simulink model "power_3pfault_generate_testdata"  (R2017b)
settings: Solver=FixedStepDiscrete  StartTime=0.0  StopTime=0.2  FixedStep=Ts  RelTol=1e-4  EnableMultiTasking=on
PreLoadFcn:
  | Ts=50e-6;
InitFcn:
  | Ts=50e-6;
undefined symbols (not defined in the file or in its folder): D1, Delta
libraries: powerlib x23
Description:
  | Copyright 2008-2017 The MathWorks, Inc.
settings Model: ExtModeTrigMode=oneshot  ExtModeArmWhenConnect=off  ExtModeAutoUpdateStatusClock=off  Creator=MathWorks  LastModifiedBy=estheim
settings DataIOCC: SaveFormat=Array  SignalLoggingSaveFormat=ModelDataLogs  SignalLoggingName=sigsOut
settings OptimizationCC: BlockReduction=off  BooleanDataType=off  ExpressionDepthLimit=2147483647  InitFltsAndDblsToZero=on  EfficientMapNaN2IntZero=off  LifeSpan=inf
settings DebuggingCC: UnderspecifiedInitializationDetection=Classic  MergeDetectMultiDrivingBlocksExec=none  CheckExecutionContextPreStartOutputMsg=on  CheckExecutionContextRuntimeOutputMsg=on  SignalResolutionControl=TryResolveAllWithWarning  MultiTaskDSMMsg=warning  MultiTaskCondExecSysMsg=none  FcnCallInpInsideContextMsg=warning  UnconnectedInputMsg=none  UnconnectedOutputMsg=none  StateNameClashWarn=warning  SFUnexpectedBacktrackingDiag=warning  SFNoUnconditionalDefaultTransitionDiag=warning  SFExecutionAtInitializationDiag=none
settings HardwareCC: ProdBitPerPointer=32  ProdBitPerSizeT=32  ProdBitPerPtrDiffT=32  ProdLargestAtomicFloat=None  ProdIntDivRoundTo=Undefined  ProdEndianess=Unspecified  ProdWordSize=32  ProdHWDeviceType=Specified  TargetUnknown=on
settings ModelReferenceCC: PropagateSignalLabelsOutOfModel=off
settings CodeAppCC: StateflowObjectComments=on
settings GRTTargetCC: TargetLangStandard=C89/C90 (ANSI)  GeneratePreprocessorConditionals=Disable all  CombineOutputUpdateFcns=off  GRTInterface=on
settings ConfigComp: CovMetricSettings=dw  CovHtmlReporting=on  CovSaveCumulativeToWorkspaceVar=on  CovSaveSingleToWorkspaceVar=on  CovExternalEMLEnable=off  CovSFcnEnable=off
settings SimscapeCC: SimscapeNormalizeSystem=off

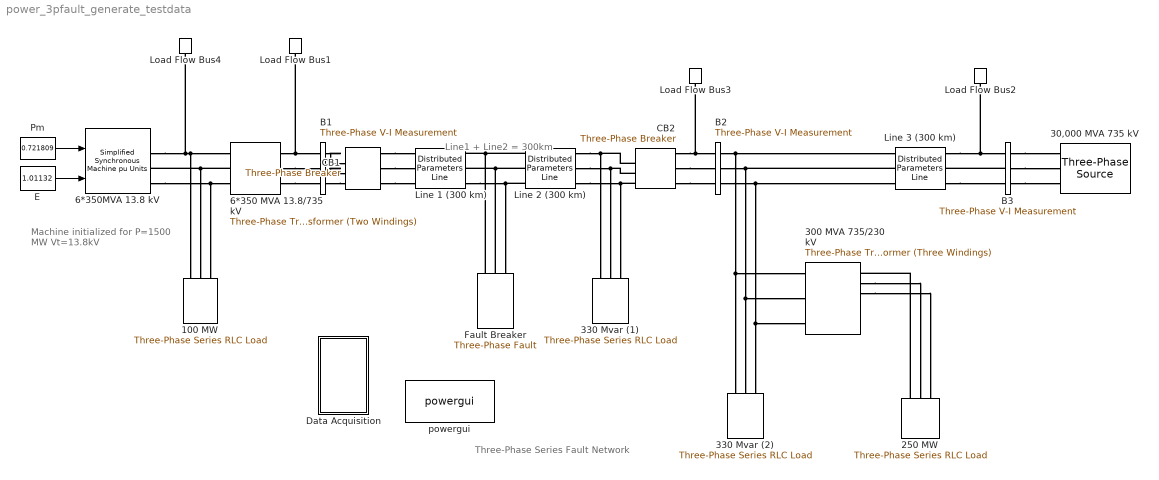
== system power_3pfault_generate_testdata ==
  note: Line1 + Line2 = 300km
  note: Machine initialized for
      |  P=1500 MW
      |  Vt=13.8kV
  note: Three-Phase Series Fault Network
  100 MW : powerlib/Elements/Three-Phase Series RLC Load  LConnTagsString=A|B|C  Configuration=Y (grounded)  NominalVoltage=13.8e3  Vabc=[1e3 1e3 1e3]  Vabcp=[1e3 1e3 1e3]  NominalFrequency=60  UnbalancedPower=off  ActivePower=100000000  InductivePower=0  CapacitivePower=0  Pabc=[10e3 9e3 11e3]  QLabc=[100 90 110]  QCabc=[100 90 110]  Pabcp=[10e3 9e3 11e3]  QLabcp=[100 90 110]  QCabcp=[100 90 110]  Measurements=None  LoadType=constant Z
  250 MW : powerlib/Elements/Three-Phase Series RLC Load  LConnTagsString=A|B|C  Configuration=Y (grounded)  NominalVoltage=230e3  Vabc=[1e3 1e3 1e3]  Vabcp=[1e3 1e3 1e3]  NominalFrequency=60  UnbalancedPower=off  ActivePower=250000000  InductivePower=0  CapacitivePower=0  Pabc=[10e3 9e3 11e3]  QLabc=[100 90 110]  QCabc=[100 90 110]  Pabcp=[10e3 9e3 11e3]  QLabcp=[100 90 110]  QCabcp=[100 90 110]  Measurements=None  LoadType=constant Z
  30,000 MVA 735 kV : powerlib/Electrical Sources/Three-Phase Source  InternalConnection=Yg  VoltagePhases=off  Voltage=(735000)*0.98865  PhaseAngle=-2.0892  Voltage_phases=[25e3 25e3 25e3]/sqrt(3)  PhaseAngles_phases=[0 -120 +120]  Frequency=60  NonIdealSource=on  SpecifyImpedance=on  Resistance=735^2/30000/10  Inductance=735^2/30000/377  ShortCircuitLevel=30000e6  BaseVoltage=735e3  XRratio=10  BusType=swing  Pref=0  Qref=0  Prefabc=[10e3, 10e3, 10e3]  Qrefabc=[0, 0, 0]  Qmin=-Inf  Qmax=Inf
  300 MVA 735/230 kV : powerlib/Elements/Three-Phase Transformer (Three Windings)  Winding1Connection=Yg  Winding2Connection=Yg  Winding3Connection=Delta (D1)  CoreType=Three single-phase transformers  SetSaturation=on  Hysteresis=off  DataFile='hysteresis'  SetInitialFlux=off  Measurements=None  UNITS=pu  NominalPower=[ 300e6 , 60 ]  Winding1=[ 735e3 , 0.002 , 0.15 ]  Winding2=[ 230e3 , 0.002 , 0 ]  Winding3=[ 25e3 , 0.05 , 0.20 ]  Rm=500  Lm=1000  L0=0.5  Saturation="[  0,0  ;  0.0012,1.2  ;  1.0,1.45 ]"  InitialFluxes=[-1.00775342585712 0.407388050044642 0.600365375812479]  MoreParameters=on  BreakLoop=on  DataType=off  TransfoNumber=0
      settings: AttributesFormatString=\n  SourceProductName=Simscape Power Systems  SourceProductBaseCode=PS
  330 Mvar (1) : powerlib/Elements/Three-Phase Series RLC Load  LConnTagsString=A|B|C  Configuration=Y (grounded)  NominalVoltage=735e3  Vabc=[1e3 1e3 1e3]  Vabcp=[1e3 1e3 1e3]  NominalFrequency=60  UnbalancedPower=off  ActivePower=1320000  InductivePower=330e6  CapacitivePower=0  Pabc=[10e3 9e3 11e3]  QLabc=[100 90 110]  QCabc=[100 90 110]  Pabcp=[10e3 9e3 11e3]  QLabcp=[100 90 110]  QCabcp=[100 90 110]  Measurements=None  LoadType=constant Z
  "330 Mvar (2) " : powerlib/Elements/Three-Phase Series RLC Load  LConnTagsString=A|B|C  Configuration=Y (grounded)  NominalVoltage=735e3  Vabc=[1e3 1e3 1e3]  Vabcp=[1e3 1e3 1e3]  NominalFrequency=60  UnbalancedPower=off  ActivePower=1320000  InductivePower=330e6  CapacitivePower=0  Pabc=[10e3 9e3 11e3]  QLabc=[100 90 110]  QCabc=[100 90 110]  Pabcp=[10e3 9e3 11e3]  QLabcp=[100 90 110]  QCabcp=[100 90 110]  Measurements=None  LoadType=constant Z
  6*350 MVA 13.8/735 kV : powerlib/Elements/Three-Phase Transformer (Two Windings)  Winding1Connection=Delta (D1)  Winding2Connection=Yg  CoreType=Three single-phase transformers  SetSaturation=off  Hysteresis=off  DataFile='hysteresis'  SetInitialFlux=off  Measurements=None  UNITS=pu  NominalPower=[ 6*350e6 , 60 ]  Winding1=[ 13.8e3 , 0.002 , 0.08 ]  Winding2=[ 735e3 , 0.002 , 0.08 ]  Rm=500  Lm=500  L0=0.5  Saturation=[ 0,0 ; 0.0024,1.2 ; 1.0,1.52 ]  InitialFluxes=[ 0.8 , -0.8 , 0.7 ]  MoreParameters=off  BreakLoop=off  DataType=off  TransfoNumber=0
  6*350MVA 13.8 kV : powerlib/Machines/Simplified Synchronous Machine pu Units  ConnectionType=3-wire Y  MechanicalLoad=Mechanical power Pm  MeasurementBus=off  NominalParameters="[ 6*350e6 13.8e3  60 ]"  Mechanical=[ inf,0,2 ]  InternalRL="[ 0.22/15  0.22 ]"  InitialConditions=[0 1.43122 0.716215 0.716215 0.716215 -3.34575 -123.346 116.654 ]  Units=0  LoadFlowParameters=[1,0,0,0,0]  TsPowergui=0  TsBlock=-1  BusType=PV  Pref=1500000000  Qref=0  Qmin=-Inf  Qmax=Inf  PLF=0  QLF=0
      settings: AttributesFormatString=\n  SourceProductName=Simscape Power Systems  SourceProductBaseCode=PS
  B1 : powerlib/Measurements/Three-Phase V-I Measurement  VoltageMeasurement=phase-to-ground  SetLabelV=on  LabelV=Vabc_B1  Vpu=on  VpuLL=off  CurrentMeasurement=yes  SetLabelI=on  LabelI=Iabc_B1  Ipu=on  Pbase=100e6  Vbase=735e3  OutputType=Complex  PhasorSimulation=off  PSBequivalent=0
  B2 : powerlib/Measurements/Three-Phase V-I Measurement  VoltageMeasurement=phase-to-ground  SetLabelV=on  LabelV=Vabc_B2  Vpu=on  VpuLL=off  CurrentMeasurement=yes  SetLabelI=on  LabelI=Iabc_B2  Ipu=on  Pbase=100e6  Vbase=735e3  OutputType=Complex  PhasorSimulation=off  PSBequivalent=0
  B3 : powerlib/Measurements/Three-Phase V-I Measurement  VoltageMeasurement=no  SetLabelV=on  LabelV=Vabc_B3  Vpu=on  VpuLL=off  CurrentMeasurement=no  SetLabelI=on  LabelI=Iabc_B3  Ipu=on  Pbase=100e6  Vbase=735e3  OutputType=Complex  PhasorSimulation=off  PSBequivalent=0
  CB1 : powerlib/Elements/Three-Phase Breaker  InitialState=closed  SwitchA=on  SwitchB=on  SwitchC=on  SwitchTimes="[5/60  ]"  External=on  BreakerResistance=0.001  SnubberResistance=1e5  SnubberCapacitance=inf  Measurements=None
      settings: AttributesFormatString=\n
  CB2 : powerlib/Elements/Three-Phase Breaker  InitialState=closed  SwitchA=on  SwitchB=on  SwitchC=on  SwitchTimes="[1/60  5/60]"  External=on  BreakerResistance=0.001  SnubberResistance=1e5  SnubberCapacitance=inf  Measurements=None
      settings: AttributesFormatString=\n
  Data Acquisition : Subsystem  mask(Data Acquisition){}
      mask Display: disp('Scopes')
  E : Constant  Value=1.01132
  Fault Breaker : powerlib/Elements/Three-Phase Fault  InitialStates=0  FaultA=off  FaultB=off  FaultC=off  GroundFault=off  SwitchTimes=[ 1/60 6/60]  External=off  SwitchStatus=NaN  FaultResistance=faultres  GroundResistance=1  SnubberResistance=inf  SnubberCapacitance=inf  Measurements=Fault voltages and currents
  Line 1 (300 km) : powerlib/Elements/Distributed Parameters Line  Phases=3  Frequency=60  Resistance=[0.01273 0.3864]  Inductance="[0.9337e-3  4.1264e-3]"  Capacitance=[12.74e-9 7.751e-9]  Length=line1  x1=[-0.001 -3.83523061350147e-08 0 0;-0.00095 -3.85597226565474e-08 0 0;-0.0009 -3.87534390922268e-08 0 0;-0.00085 -3.89333866155258e-08 0 0;-0.0008 -3.90995012919463e-08 0 0;-0.00075 -3.92517241017346e-08 0 0;-0.0007 -3.93900009608513e-08 0 0;-0.00065 -3.95142827401867e-08 0 0;-0.0006 -3.96245252830165e-08 569012.028774079 -563710.851617423;-0.00055 -3.97206894206901e-08 579536.036921589 -552885.768257326;-0.0005 -3.98027409865472e-08 589854.138674711 -541864.247216397;-0.00045 -3.98706508280573e-08 599962.668061021 -530650.204388584;-0.0004 -3.9924394817177e-08 609858.033568162 -519247.624069904;-0.00035 -3.99639538589228e-08 619536.719419888 -507660.557542852;-0.0003 -3.99893138981557e-08 628995.286825201 -495893.12163699;-0.00025 -4.00004659245744e-08 638230.37520014 -483949.497266264;-0.0002 -3.9997405975917e-08 647238.703361779 -471833.927943542;-0.00015 -3.99801351393688e-08 656017.070694018 -459550.718272915;-0.0001 -3.99486595511756e-08 664562.358284742 -447104.23242029;-5e-05 -3.99029903944642e-08 672871.53003396 -434498.892562826]  x2=[-0.001 -2.553918458856e-08 0 0;-0.00095 -2.56957373164155e-08 0 0;-0.0009 -2.58431604711559e-08 0 0;-0.00085 -2.59814016740361e-08 0 0;-0.0008 -2.6110411808615e-08 0 0;-0.00075 -2.62301450382062e-08 0 0;-0.0007 -2.63405588221631e-08 0 0;-0.00065 -2.64416139309943e-08 0 0;-0.0006 -2.65332744603006e-08 471233.93631822 -623559.418978757;-0.00055 -2.66155078435325e-08 482903.361814212 -614566.656381502;-0.0005 -2.66882848635605e-08 494401.214045154 -605355.541177567;-0.00045 -2.67515796630559e-08 505723.407878895 -595929.346032323;-0.0004 -2.68053697536778e-08 516865.920593878 -586291.420028021;-0.00035 -2.68496360240632e-08 527824.793308393 -576445.187473879;-0.0003 -2.68843627466169e-08 538596.132387145 -566394.14668944;-0.00025 -2.69095375830998e-08 549176.110824649 -556141.868761635;-0.0002 -2.69251515890124e-08 559560.969604944 -545691.996275993;-0.00015 -2.69311992167726e-08 569747.019037153 -535048.242022452;-0.0001 -2.69276783176873e-08 579730.640066417 -524214.387676215;-5e-05 -2.6914590142715e-08 589508.285559721 -513194.282454146]  x3=[-0.001 -4.49470039159052e-11 0 0;-0.00095 -4.45017594860336e-11 0 0;-0.0009 -4.40407037929171e-11 0 0;-0.00085 -4.35640006474479e-11 0 0;-0.0008 -4.30718194199839e-11 0 0;-0.00075 -4.25643349801714e-11 0 0;-0.0007 -4.20417276348157e-11 0 0;-0.00065 -4.15041830638179e-11 0 0;-0.0006 -4.09518922542046e-11 797.412721573975 -699.30782653233;-0.00055 -4.03850514322706e-11 810.451823819326 -684.153849460542;-0.0005 -3.9803861993861e-11 823.202976390736 -668.756795783721;-0.00045 -3.92085304328157e-11 835.661648864413 -653.122136001722;-0.0004 -3.85992682676037e-11 847.82341473335 -637.25542503472;-0.00035 -3.79762919661712e-11 859.683952980043 -621.16230024957;-0.0003 -3.73398228690317e-11 871.239049611729 -604.848479456878;-0.00025 -3.66900871106248e-11 882.484599157596 -588.319758879493;-0.0002 -3.60273155389717e-11 893.416606127436 -571.582011093132;-0.00015 -3.53517436336559e-11 904.031186431228 -554.641182939885;-0.0001 -3.46636114221585e-11 914.324568759132 -537.503293415329;-5e-05 -3.39631633945778e-11 924.293095921421 -520.174431530008]  x4=[-0.001 -3.11690622475258e-11 0 0;-0.00095 -3.23804662907721e-11 0 0;-0.0009 -3.35803657085288e-11 0 0;-0.00085 -3.47683341822461e-11 0 0;-0.0008 -3.5943949632382e-11 0 0;-0.00075 -3.71067943683649e-11 0 0;-0.0007 -3.8256455236997e-11 0 0;-0.00065 -3.93925237692461e-11 0 0;-0.0006 -4.05145963253721e-11 2537.32214813318 -4084.70327813382;-0.00055 -4.16222742383388e-11 2613.86195927345 -4036.15312731875;-0.0005 -4.27151639554579e-11 2689.4730777058 -3986.16895051616;-0.00045 -4.37928771782169e-11 2764.12863915988 -3934.76850686606;-0.0004 -4.48550310002395e-11 2837.80211887019 -3881.97005870134;-0.00035 -4.59012480433302e-11 2910.4673410002 -3827.79236505922;-0.0003 -4.69311565915554e-11 2982.09848794249 -3772.25467501628;-0.00025 -4.79443907233118e-11 3052.67010949162 -3715.37672084934;-0.0002 -4.89405904413371e-11 3122.1571318865 -3657.17871102469;-0.00015 -4.99194018006149e-11 3190.53486671894 -3597.6813230181;-0.0001 -5.08804770341302e-11 3257.77901970535 -3536.90569596823;-5e-05 -5.18234746764286e-11 3323.86569931835 -3474.87342316597]  x5=0.000961420663892762  V1=ones(3,3)  V2=ones(3,3)  I1=ones(3,3)  I2=ones(3,3)  nHarmo=1  Measurements=None
      settings: AttributesFormatString=\n  SourceProductName=Simscape Power Systems
  Line 2 (300 km) : powerlib/Elements/Distributed Parameters Line  Phases=3  Frequency=60  Resistance=[0.01273 0.3864]  Inductance="[0.9337e-3  4.1264e-3]"  Capacitance=[12.74e-9 7.751e-9]  Length=line2  x1=[-0.00075 -2.62301450382062e-08 435237.977089234 -649196.034954563;-0.0007 -2.63405588221631e-08 447397.009382411 -640877.184725142;-0.00065 -2.64416139309943e-08 459397.083648489 -632330.633883601;-0.0006 -2.65332744603006e-08 471233.93631822 -623559.418978757;-0.00055 -2.66155078435325e-08 482903.361814212 -614566.656381502;-0.0005 -2.66882848635605e-08 494401.214045154 -605355.541177567;-0.00045 -2.67515796630559e-08 505723.407878895 -595929.346032323;-0.0004 -2.68053697536778e-08 516865.920593878 -586291.420028021;-0.00035 -2.68496360240632e-08 527824.793308393 -576445.187473879;-0.0003 -2.68843627466169e-08 538596.132387145 -566394.14668944;-0.00025 -2.69095375830998e-08 549176.110824649 -556141.868761635;-0.0002 -2.69251515890124e-08 559560.969604944 -545691.996275993;-0.00015 -2.69311992167726e-08 569747.019037153 -535048.242022452;-0.0001 -2.69276783176873e-08 579730.640066417 -524214.387676215;-5e-05 -2.6914590142715e-08 589508.285559721 -513194.282454146]  x2=[-0.00075 -1.34555410810238e-08 344174.875497498 -668903.306709846;-0.0007 -1.34994132809944e-08 356721.531395338 -662297.342990336;-0.00065 -1.35384892037052e-08 369141.445831646 -655456.068178468;-0.0006 -1.35727549656671e-08 381430.206069961 -648381.912946609;-0.00055 -1.3602198392418e-08 393583.445972283 -641077.390708426;-0.0005 -1.36268090228485e-08 405596.847550346 -633545.09672589;-0.00045 -1.36465781129189e-08 417466.142499771 -625787.707187188;-0.0004 -1.36614986387655e-08 429187.113716581 -617807.978255883;-0.00035 -1.36715652991966e-08 440755.596795512 -609608.745091671;-0.0003 -1.36767745175757e-08 452167.481509611 -601192.92084305;-0.00025 -1.36771244430923e-08 463418.713270579 -592563.495612306;-0.0002 -1.36726149514195e-08 474505.294569345 -583723.535393131;-0.00015 -1.36632476447582e-08 485423.286396363 -574676.1809813;-0.0001 -1.36490258512679e-08 496168.809641125 -565424.646858755;-5e-05 -1.36299546238841e-08 506738.046470388 -555972.220051516]  x3=[-0.00075 -3.5871254563586e-11 895.394930749455 -547.480315802248;-0.0007 -3.49539952778335e-11 905.554875500122 -530.506479933979;-0.00065 -3.40243170039963e-11 915.393080915431 -513.344157639458;-0.0006 -3.30825500523384e-11 924.906051527842 -495.999446610078;-0.00055 -3.21290290281733e-11 934.090407424195 -478.478509339076;-0.0005 -3.11640927129808e-11 942.942885446572 -460.787570932038;-0.00045 -3.01880839440388e-11 951.460340351683 -442.932916895143;-0.0004 -2.92013494926156e-11 959.639745928359 -424.920890901952;-0.00035 -2.82042399407633e-11 967.478196072744 -406.757892539535;-0.0003 -2.71971095567579e-11 974.972905820825 -388.450375034723;-0.00025 -2.61803161692293e-11 982.121212337917 -370.004842961315;-0.0002 -2.51542210400264e-11 988.920575864752 -351.427849929024;-0.00015 -2.41191887358627e-11 995.368580619844 -332.725996255018;-0.0001 -2.30755869987876e-11 1001.46293565781 -313.905926618857;-5e-05 -2.20237866155289e-11 1007.20147568331 -294.974327701669]  x4=[-0.00075 -1.46274524402325e-11 1559.23654654393 -4542.2395601569;-0.0007 -1.59066397662847e-11 1644.57396066192 -4512.04345417997;-0.00065 -1.71801755389692e-11 1729.32706548251 -4480.24424064839;-0.0006 -1.84476072770902e-11 1813.46574863114 -4446.85321767132;-0.00055 -1.97084846681861e-11 1896.9601160343 -4411.88224892023;-0.0005 -2.09623597285237e-11 1979.78050254084 -4375.3437594138;-0.00045 -2.22087869622644e-11 2061.89748246179 -4337.25073110336;-0.0004 -2.34473235197473e-11 2143.28188002518 -4297.61669826049;-0.00035 -2.46775293548307e-11 2223.90477974209 -4256.45574266834;-0.0003 -2.58989673812394e-11 2303.73753668015 -4213.78248861844;-0.00025 -2.71112036278585e-11 2382.75178664094 -4169.61209771475;-0.0002 -2.83138073929218e-11 2460.91945623769 -4123.96026348684;-0.00015 -2.95063513970379e-11 2538.21277286959 -4076.84320581404;-0.0001 -3.06884119350007e-11 2614.6042745893 -4028.27766516259;-5e-05 -3.18595690263294e-11 2690.06681985999 -3978.28089663782]  x5=0.000735204037094465  V1=ones(3,3)  V2=ones(3,3)  I1=ones(3,3)  I2=ones(3,3)  nHarmo=1  Measurements=None
      settings: AttributesFormatString=\n  SourceProductName=Simscape Power Systems
  Line 3 (300 km) : powerlib/Elements/Distributed Parameters Line  Phases=3  Frequency=60  Resistance=[0.01273 0.3864]  Inductance="[0.9337e-3  4.1264e-3]"  Capacitance=[12.74e-9 7.751e-9]  Length=300  x1=[-0.0017 -1.17416070170318e-08 0 0;-0.00165 -1.18731208257341e-08 0 0;-0.0016 -1.20004161711422e-08 0 0;-0.00155 -1.21234478258262e-08 0 0;-0.0015 -1.22421720772248e-08 0 0;-0.00145 -1.23565467431769e-08 0 0;-0.0014 -1.24665311869084e-08 0 0;-0.00135 -1.257208633147e-08 0 0;-0.0013 -1.26731746736215e-08 0 0;-0.00125 -1.27697602971563e-08 0 0;-0.0012 -1.28618088856622e-08 0 0;-0.00115 -1.29492877347141e-08 0 0;-0.0011 -1.30321657634934e-08 0 0;-0.00105 -1.31104135258311e-08 266485.469647642 -703470.130718914;-0.001 -1.31840032206698e-08 279697.460285226 -698322.348619587;-0.00095 -1.32529087019415e-08 292810.075746983 -692926.45591494;-0.0009 -1.33171054878566e-08 305818.657183077 -687284.369739957;-0.00085 -1.33765707696029e-08 318718.582706466 -681398.094700991;-0.0008 -1.34312834194489e-08 331505.269035035 -675269.722163535;-0.00075 -1.34812239982505e-08 344174.173120017 -668901.429509172;-0.0007 -1.3526374762358e-08 356720.793760116 -662295.479361956;-0.00065 -1.35667196699199e-08 369140.67320076 -655454.218784522;-0.0006 -1.36022443865826e-08 381429.398717923 -648380.078444176;-0.00055 -1.36329362905835e-08 393582.604185942 -641075.571749297;-0.0005 -1.36587844772351e-08 405595.971628784 -633543.293956332;-0.00045 -1.36797797627999e-08 417465.2327542 -625785.921247716;-0.0004 -1.36959146877529e-08 429186.170470228 -617806.209781034;-0.00035 -1.3707183519432e-08 440754.620383508 -609606.994709774;-0.0003 -1.3713582254075e-08 452166.472278871 -601191.189176009;-0.00025 -1.3715108618242e-08 463417.671579678 -592561.783275373;-0.0002 -1.3711762069623e-08 474504.22078839 -583721.842994692;-0.00015 -1.37035437972309e-08 485422.180906864 -574674.509122656;-0.0001 -1.36904567209786e-08 496167.672835857 -565422.996133909;-5e-05 -1.36725054906422e-08 506736.878753252 -555970.591046963]  x2=[-0.0017 -5.98477587943826e-10 0 0;-0.00165 -5.98573183271785e-10 0 0;-0.0016 -5.98456108397903e-10 0 0;-0.00155 -5.98126404918327e-10 0 0;-0.0015 -5.97584189975134e-10 0 0;-0.00145 -5.96829656214709e-10 0 0;-0.0014 -5.95863071719307e-10 0 0;-0.00135 -5.94684779911795e-10 0 0;-0.0013 -5.93295199433642e-10 0 0;-0.00125 -5.91694823996175e-10 0 0;-0.0012 -5.89884222205168e-10 0 0;-0.00115 -5.87864037358814e-10 0 0;-0.0011 -5.8563498721917e-10 0 0;-0.00105 -5.83197863757138e-10 96636.3853033394 -730540.783651741;-0.001 -5.80553532871078e-10 110388.774729698 -728589.563067858;-0.00095 -5.77702934079163e-10 124101.943550024 -726379.478081482;-0.0009 -5.74647080185571e-10 137771.019540733 -723911.313925286;-0.00085 -5.71387056920639e-10 151391.146144212 -721185.94752624;-0.0008 -5.67924022555109e-10 164957.484194333 -718204.347194051;-0.00075 -5.64259207488603e-10 178465.213635784 -714967.572277119;-0.0007 -5.60393913812464e-10 191909.535236613 -711476.772786159;-0.00065 -5.56329514847128e-10 205285.672293373 -707733.188985608;-0.0006 -5.52067454654196e-10 218588.872328259 -703738.150952967;-0.00055 -5.47609247523359e-10 231814.408777643 -699493.078106223;-0.0005 -5.42956477434384e-10 244957.582671401 -694999.478699548;-0.00045 -5.38110797494327e-10 258013.724302429 -690258.949287412;-0.0004 -5.33073929350199e-10 270978.194885776 -685273.174157345;-0.00035 -5.27847662577267e-10 283846.388206775 -680043.924731508;-0.0003 -5.2243385404323e-10 296613.732257611 -674573.058937323;-0.00025 -5.16834427248483e-10 309275.690861738 -668862.520547358;-0.0002 -5.11051371642702e-10 321827.765285555 -662914.338488709;-0.00015 -5.05086741918007e-10 334265.495836786 -656730.626122141;-0.0001 -4.9894265727894e-10 346584.463448991 -650313.580491212;-5e-05 -4.92621300689515e-10 358780.291251636 -643665.481541679]  x3=[-0.0017 -2.08055981742597e-11 0 0;-0.00165 -2.057063726502e-11 0 0;-0.0016 -2.03283677063097e-11 0 0;-0.00155 -2.00788755753492e-11 0 0;-0.0015 -1.98222495155047e-11 0 0;-0.00145 -1.95585807047934e-11 0 0;-0.0014 -1.92879628234881e-11 0 0;-0.00135 -1.90104920208336e-11 0 0;-0.0013 -1.87262668808847e-11 0 0;-0.00125 -1.84353883874804e-11 0 0;-0.0012 -1.81379598883643e-11 0 0;-0.00115 -1.78340870584659e-11 0 0;-0.0011 -1.75238778623548e-11 0 0;-0.00105 -1.72074425158812e-11 146.085371214708 -1136.76931922377;-0.001 -1.68848934470169e-11 167.485631246302 -1133.81409432616;-0.00095 -1.65563452559103e-11 188.826384430616 -1130.45603067962;-0.0009 -1.62219146741693e-11 210.100048499661 -1126.69632138818;-0.00085 -1.58817205233872e-11 231.299065021891 -1122.53630225865;-0.0008 -1.55358836729257e-11 252.415902087675 -1117.97745132602;-0.00075 -1.51845269969712e-11 273.443056985357 -1113.02138832831;-0.0007 -1.48277753308776e-11 294.373058866922 -1107.66987413112;-0.00065 -1.44657554268132e-11 315.198471402365 -1101.92481010194;-0.0006 -1.4098595908726e-11 335.911895421773 -1095.78823743468;-0.00055 -1.37264272266445e-11 356.505971544221 -1089.26233642439;-0.0005 -1.33493816103294e-11 376.973382792526 -1082.34942569261;-0.00045 -1.29675930222929e-11 397.306857192927 -1075.05196136362;-0.0004 -1.25811971102022e-11 417.499170358791 -1067.37253619175;-0.00035 -1.21903311586852e-11 437.543148057398 -1059.31387864018;-0.0003 -1.17951340405531e-11 457.431668758914 -1050.87885191159;-0.00025 -1.13957461674604e-11 477.157666166635 -1042.07045293079;-0.0002 -1.09923094400166e-11 496.714131727609 -1032.89181128001;-0.00015 -1.05849671973699e-11 516.094117122743 -1023.34618808691;-0.0001 -1.01738641662795e-11 535.290736735507 -1013.43697486597;-5e-05 -9.75914640969494e-12 554.297170098358 -1003.16769231347]  x4=[-0.0017 7.46115628674393e-12 0 0;-0.00165 6.97035919471124e-12 0 0;-0.0016 6.47708556724684e-12 0 0;-0.00155 5.98151066212182e-12 0 0;-0.0015 5.4838105547402e-12 0 0;-0.00145 4.9841620755803e-12 0 0;-0.0014 4.48274274736762e-12 0 0;-0.00135 3.97973072200191e-12 0 0;-0.0013 3.47530471726063e-12 0 0;-0.00125 2.96964395330138e-12 0 0;-0.0012 2.46292808898584e-12 0 0;-0.00115 1.9553371580478e-12 0 0;-0.0011 1.44705150512807e-12 0 0;-0.00105 9.38251721698883e-13 141.894515453802 -4366.94257638276;-0.001 4.29118581900568e-13 224.179568795925 -4363.4921905219;-0.00095 -8.01670216865948e-14 306.384972204712 -4358.49147666302;-0.0009 -5.89424142312681e-13 388.481518491763 -4351.94221153596;-0.00085 -1.09847184334761e-12 470.440039145095 -4343.84672206343;-0.0008 -1.60712926256711e-12 552.231414692574 -4334.20788453429;-0.00075 -2.11521567641215e-12 633.826585047928 -4323.02912358161;-0.0007 -2.62255056419921e-12 715.196559835654 -4310.31441096594;-0.00065 -3.12895367225839e-12 796.312428691164 -4296.06826416412;-0.0006 -3.63424507797671e-12 877.145371532495 -4280.29574476429;-0.00055 -4.1382452537237e-12 957.666668799952 -4263.00245666747;-0.0005 -4.64077513063679e-12 1037.84771166003 -4244.19454409658;-0.00045 -5.14165616224357e-12 1117.66001216998 -4223.87868941341;-0.0004 -5.6407103878985e-12 1197.07521339949 -4202.06211074439;-0.00035 -6.13776049601152e-12 1276.06509950568 -4178.75255941604;-0.0003 -6.63262988704597e-12 1354.60160575816 -4153.95831720095;-0.00025 -7.12514273626361e-12 1432.65682851021 -4127.68819337532;-0.0002 -7.61512405619426e-12 1510.20303511285 -4099.95152158906;-0.00015 -8.10239975880806e-12 1587.21267376813 -4070.75815654958;-0.0001 -8.58679671736809e-12 1663.65838331811 -4040.11847052048;-5e-05 -9.06814282794148e-12 1739.51300296621 -4008.0433496363]  x5=0.00169662470098723  V1=ones(3,3)  V2=ones(3,3)  I1=ones(3,3)  I2=ones(3,3)  nHarmo=1  Measurements=None
      settings: AttributesFormatString=\n  SourceProductName=Simscape Power Systems
  Load Flow Bus1 : powerlib/Measurements/Load Flow Bus  LConnTagsString=a  Phases=single  Connectors=on one side  ID=B1  Vbase=735e3  Vref=1  Vangle=0  VLF=1.012  VLFb=1  VLFc=1  angleLF=16.39  angleLFb=0  angleLFc=0
      settings: AttributesFormatString=%<ID>\n%<Vbase>V\n%<VLF>pu\n%<angleLF>deg.  SourceProductName=Simscape Power Systems
  Load Flow Bus2 : powerlib/Measurements/Load Flow Bus  LConnTagsString=a  Phases=single  Connectors=on one side  ID=B3  Vbase=735e3  Vref=1  Vangle=0  VLF=1  VLFb=1  VLFc=1  angleLF=0  angleLFb=0  angleLFc=0
      settings: AttributesFormatString=%<ID>\n%<Vbase>V\n%<VLF>pu\n%<angleLF>deg.  SourceProductName=Simscape Power Systems
  Load Flow Bus3 : powerlib/Measurements/Load Flow Bus  LConnTagsString=a  Phases=single  Connectors=on one side  ID=B2  Vbase=735e3  Vref=1  Vangle=0  VLF=1.03  VLFb=1  VLFc=1  angleLF=7.354  angleLFb=0  angleLFc=0
      settings: AttributesFormatString=%<ID>\n%<Vbase>V\n%<VLF>pu\n%<angleLF>deg.  SourceProductName=Simscape Power Systems
  Load Flow Bus4 : powerlib/Measurements/Load Flow Bus  LConnTagsString=a  Phases=single  Connectors=on one side  ID=GEN  Vbase=13.8e3  Vref=1  Vangle=0  VLF=1  VLFb=1  VLFc=1  angleLF=-7.552  angleLFb=0  angleLFc=0
      settings: AttributesFormatString=%<ID>\n%<Vbase>V\n%<VLF>pu\n%<angleLF>deg.  SourceProductName=Simscape Power Systems
  Pm : Constant  Value=0.721809
  powergui : powerlib/powergui  Priority=2  SimulationMode=Discrete  SampleTime=Ts  frequency=60  Iterations=50  frequencyindice=60  Pbase=100e6  ErrMax=0.0001  UnitsV=kV  UnitsW=MW  buscounter=0  FunctionMessages=off  echomessages=off  EnableUseOfTLC=off  CurrentSourceSwitches=off  DisableSnubberDevices=off  DisableRonSwitches=off  DisableVfSwitches=off  DisplayEquations=off  SolverType=Tustin/Backward Euler (TBE)  Interpol=off  ExternalGateDelay=off  methode=off  Ts=0  x0status=blocks  SPID=off  SwTol=0  HookPort=off  RestoreLinks=warning  ResistiveCurrentMeasurement=off  Frange=0:0.5:500  Ylog=off  Xlog=off  ShowGrid=off  save=on  variable=Zmes  structure=0  ZoomFFT=on  StartTime=0.0  cycles=1  DisplayStyle=off  fundamental=60  FreqAxis=off  MaxFrequency=1000  frequencyindicesteady=1  RmsSteady=1  display=off
  wires:
  Pm/1 -> 6*350MVA 13.8 kV/1
  E/1 -> 6*350MVA 13.8 kV/2
  connections:
  6*350 MVA 13.8/735 kV/LConn2 -- 6*350MVA 13.8 kV/RConn2 -- 100 MW/LConn2
  6*350MVA 13.8 kV/RConn1 -- 6*350 MVA 13.8/735 kV/LConn1 -- 100 MW/LConn1 -- Load Flow Bus4/LConn1
  6*350MVA 13.8 kV/RConn3 -- 6*350 MVA 13.8/735 kV/LConn3 -- 100 MW/LConn3
  6*350 MVA 13.8/735 kV/RConn2 -- B1/LConn2
  6*350 MVA 13.8/735 kV/RConn1 -- B1/LConn1 -- Load Flow Bus1/LConn1
  6*350 MVA 13.8/735 kV/RConn3 -- B1/LConn3
  B1/RConn2 -- CB1/LConn2
  B1/RConn1 -- CB1/LConn1
  B1/RConn3 -- CB1/LConn3
  CB1/RConn2 -- Line 1 (300 km)/LConn2
  CB1/RConn1 -- Line 1 (300 km)/LConn1
  CB1/RConn3 -- Line 1 (300 km)/LConn3
  CB2/LConn1 -- Line 2 (300 km)/RConn1 -- 330 Mvar (1)/LConn1
  Line 1 (300 km)/RConn3 -- Line 2 (300 km)/LConn3 -- Fault Breaker/LConn3
  CB2/RConn2 -- B2/LConn2
  CB2/RConn1 -- B2/LConn1 -- Load Flow Bus3/LConn1
  CB2/RConn3 -- B2/LConn3
  CB2/LConn2 -- Line 2 (300 km)/RConn2 -- 330 Mvar (1)/LConn2
  B2/RConn2 -- Line 3 (300 km)/LConn2 -- "330 Mvar (2) "/LConn2 -- 300 MVA 735/230 kV/LConn2
  300 MVA 735/230 kV/RConn2 -- 250 MW/LConn2
  250 MW/LConn1 -- 300 MVA 735/230 kV/RConn1
  300 MVA 735/230 kV/RConn3 -- 250 MW/LConn3
  Line 3 (300 km)/RConn1 -- B3/LConn1 -- Load Flow Bus2/LConn1
  B3/LConn2 -- Line 3 (300 km)/RConn2
  Line 3 (300 km)/RConn3 -- B3/LConn3
  B3/RConn3 -- 30,000 MVA 735 kV/RConn3
  B3/RConn2 -- 30,000 MVA 735 kV/RConn2
  B3/RConn1 -- 30,000 MVA 735 kV/RConn1
  B2/RConn1 -- Line 3 (300 km)/LConn1 -- "330 Mvar (2) "/LConn1 -- 300 MVA 735/230 kV/LConn1
  B2/RConn3 -- Line 3 (300 km)/LConn3 -- "330 Mvar (2) "/LConn3 -- 300 MVA 735/230 kV/LConn3
  Fault Breaker/LConn1 -- Line 2 (300 km)/LConn1 -- Line 1 (300 km)/RConn1
  Fault Breaker/LConn2 -- Line 2 (300 km)/LConn2 -- Line 1 (300 km)/RConn2
  CB2/LConn3 -- Line 2 (300 km)/RConn3 -- 330 Mvar (1)/LConn3

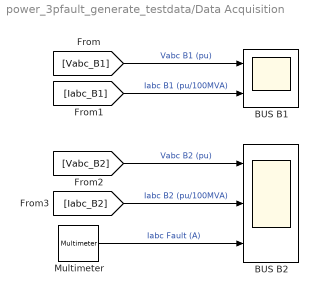
== system power_3pfault_generate_testdata/Data Acquisition ==
  BUS B1 : Scope  NumInputPorts=2
  BUS B2 : Scope  NumInputPorts=3
  Multimeter : powerlib/Measurements/Multimeter  Tag=PoWeRsYsTeMmEaSuReMeNt  PhasorSimulation=off  OutputType=Magnitude  sel=4  L=6  Gain=1  yselected={'Ib: Fault Breaker/Fault A'};  PSBOutputType=1  PSBequivalent=0  AxesSetting=[0,0.1,-100,100]  Display=0  SavedBlockNames={}
      settings: AttributesFormatString=\n
  wires:
  [Vabc_B1] -> BUS B1/1  "Vabc B1 (pu)"
  [Iabc_B1] -> BUS B1/2  "Iabc B1 (pu/100MVA)"
  [Vabc_B2] -> BUS B2/1  "Vabc B2 (pu)"
  [Iabc_B2] -> BUS B2/2  "Iabc B2 (pu/100MVA)"
  Multimeter/1 -> BUS B2/3  "Iabc Fault (A)"
